simulink model "modelcomplet"  (R2021b)
settings: Solver=ode1  StartTime=0.0  StopTime=50  FixedStep=0.01  RelTol=1e-6  EnableMultiTasking=on
values from neighbouring files (symbols this model uses):
  a = -l^2+J/(mc+mp)    (= 0.00589092533208)    [parameters.m]    (also in simulation_models.m)
  A1 = expm(A(2:4,2:4)*0.01)    [simulation_models.m]
  B1 = (A1-eye(3))*inv(A(2:4,2:4))*B(2:4)    [simulation_models.m]
  DZcp = 6.8    [parameters.m]    (also in simulation_models.m)
  DZcv = 0.08    [parameters.m]    (also in simulation_models.m)
  DZu = 0.4    [parameters.m]    (also in simulation_models.m)
  FCD = 0.2501    [parameters.m]    (also in simulation_models.m)
  FCU = 0.8793    [parameters.m]    (also in simulation_models.m)
  fp = 0.0038    [parameters.m]    (also in simulation_models.m)
  FS = 2    [parameters.m]    (also in simulation_models.m)
  FSD = 2.7457    [parameters.m]    (also in simulation_models.m)
  FSdl = -1    [parameters.m]    (also in simulation_models.m)
  FSU = 2.7972    [parameters.m]    (also in simulation_models.m)
  FSul = 2    [parameters.m]    (also in simulation_models.m)
  g = 9.81    [parameters.m]    (also in simulation_models.m)
  J = 0.0075    [parameters.m]    (also in simulation_models.m)
  l = 0.0167903    [parameters.m]    (also in simulation_models.m)
  L1 = L1'    [simulation_models.m]
  M = 22.304    [parameters.m]    (also in simulation_models.m)
  mu = l*(mc+mp)    (= 0.0204002145)    [parameters.m]    (also in simulation_models.m)
  Um = 0.5    [parameters.m]    (also in simulation_models.m)
  Xc = 2    [parameters.m]    (also in simulation_models.m)
  Yc = 2    [parameters.m]    (also in simulation_models.m)
undefined symbols (not defined in the file or in its folder): DiscIntNeverNeededParam
settings Model: Creator=szmis  LastModifiedBy=szmis
settings DataIOCC: SaveFormat=Array  SignalLoggingSaveFormat=ModelDataLogs  ReturnWorkspaceOutputs=off
settings OptimizationCC: BlockReduction=off  BooleanDataType=off
settings DebuggingCC: SaveWithParameterizedLinksMsg=none  UnderspecifiedInitializationDetection=Classic  MergeDetectMultiDrivingBlocksExec=none  SignalResolutionControl=TryResolveAllWithWarning  MultiTaskDSMMsg=warning  MultiTaskCondExecSysMsg=none
settings HardwareCC: TargetUnknown=on
settings ModelReferenceCC: PropagateSignalLabelsOutOfModel=off
settings GRTTargetCC: CombineOutputUpdateFcns=off  GRTInterface=on

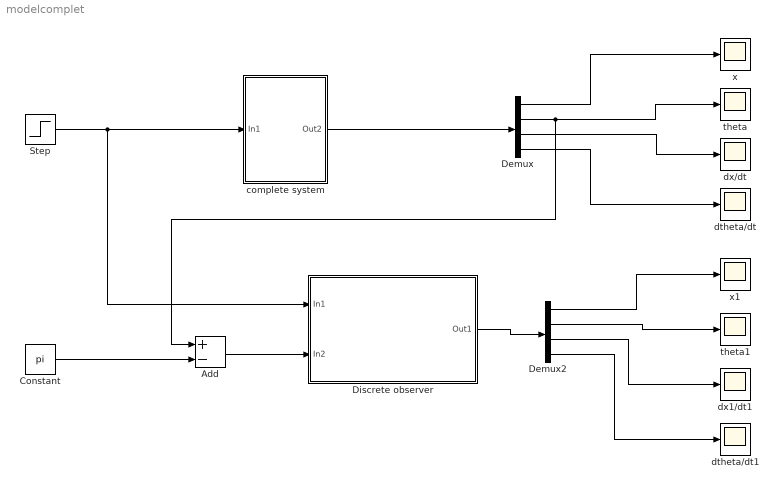
== system modelcomplet ==
  Add : Sum  Inputs=+-
  Constant : Constant  Value=pi
  Demux : Demux
  Demux2 : Demux
  Discrete observer : Subsystem
  Step : Step  After=0.3  SampleTime=0
  complete system : Subsystem
  dtheta/dt : Scope
  dtheta/dt1 : Scope
  dx/dt : Scope
  dx1/dt1 : Scope
  theta : Scope
  theta1 : Scope
  x : Scope
  x1 : Scope
  wires:
  Demux2/3 -> dx1/dt1/1
  Demux2/2 -> theta1/1
  Add/1 -> Discrete observer/2(In2)
  Demux/2 -> theta/1, Add/1
  Discrete observer/1(Out1) -> Demux2/1
  Constant/1 -> Add/2
  Demux/3 -> dx/dt/1
  Demux/1 -> x/1
  complete system/1(Out2) -> Demux/1
  Demux/4 -> dtheta/dt/1
  Demux2/1 -> x1/1
  Step/1 -> complete system/1(In1), Discrete observer/1(In1)
  Demux2/4 -> dtheta/dt1/1

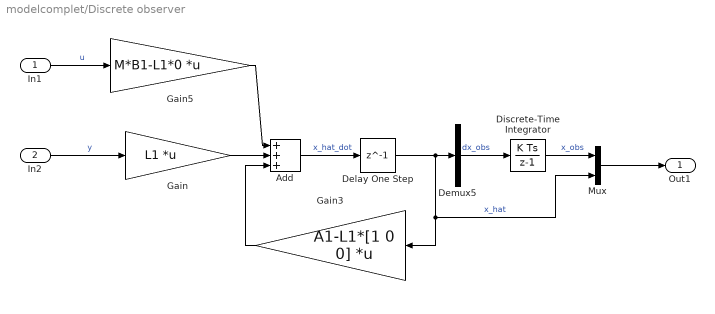
== system modelcomplet/Discrete observer ==
  In1 : Inport
  In2 : Inport  Port=2
  Add : Sum  Inputs=+++
  Delay One Step : Delay  DelayLength=1
  Demux5 : Demux  Outputs=3
  Discrete-Time Integrator : DiscreteIntegrator  SampleTime=0.01  ICPrevOutput=DiscIntNeverNeededParam  ICPrevScaledInput=DiscIntNeverNeededParam
  Gain : Gain  Gain=L1  Multiplication=Matrix(K*u)
  Gain3 : Gain  Gain=A1-L1*[1 0 0]  Multiplication=Matrix(K*u)
  Gain5 : Gain  Gain=M*B1-L1*0  Multiplication=Matrix(K*u)
  Mux : Mux  Inputs=2
  Out1 : Outport
  wires:
  In2/1 -> Gain/1  "y"
  Add/1 -> Delay One Step/1  "x_hat_dot"
  In1/1 -> Gain5/1  "u"
  Gain/1 -> Add/2
  Gain3/1 -> Add/3
  Gain5/1 -> Add/1
  Delay One Step/1 -> Demux5/1, Gain3/1, Mux/2  "x_hat"
  Mux/1 -> Out1/1
  Discrete-Time Integrator/1 -> Mux/1  "x_obs"
  Demux5/2 -> Discrete-Time Integrator/1  "dx_obs"

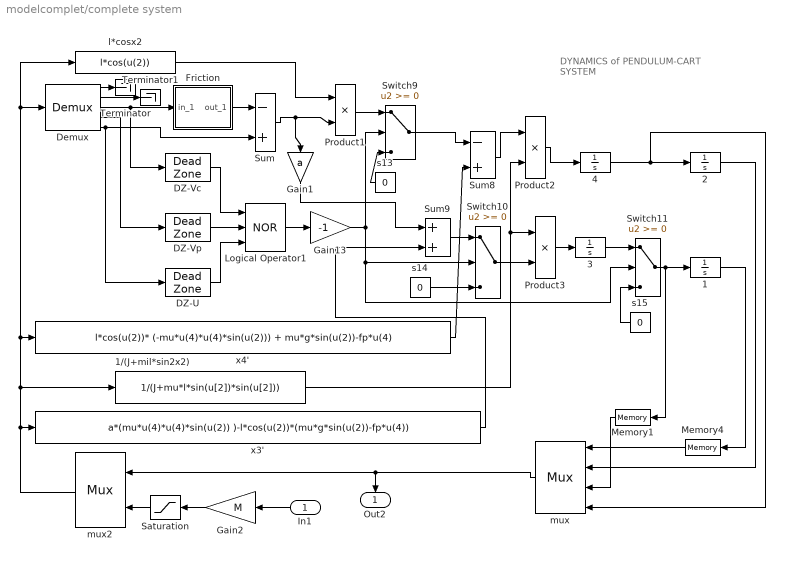
== system modelcomplet/complete system ==
  note: DYNAMICS
      | of
      | PENDULUM-CART SYSTEM
  In1 : Inport
  1 : Integrator
  1/(J+mil*sin2x2) : Fcn  Expr=1/(J+mu*l*sin(u[2])*sin(u[2]))
  2 : Integrator  InitialCondition=pi
  3 : Integrator
  4 : Integrator
  DZ-U : DeadZone  LowerValue=-DZu  UpperValue=DZu  SaturateOnIntegerOverflow=on
  DZ-Vc : DeadZone  LowerValue=-DZcv  UpperValue=DZcv  SaturateOnIntegerOverflow=on
  DZ-Vp : DeadZone  LowerValue=-DZcp  UpperValue=DZcp  SaturateOnIntegerOverflow=on
  Demux : Demux  Outputs=5
  Friction : Subsystem  mask(Friction model){FSD=FSD, FSU=FSU, FCD=FCD, FCU=FCU, FSdl=FSdl, FSul=FSul, FS=FS, Xc=Xc, Yc=Yc, small=DZcv}
      mask prompts: FSD "Static friction (FSD) [N]:"; FSU "Static friction (FSU) [N] :"; FCD "Columbic friction (FCD) [N]:"; FCU "Coulombic friction (FCU)  [N] :"; FSdl "Coulombic friction (FSdl) [N]:"; FSul "Coulombic friction (Fsul) [N]:"; FS "Coulombic friction (FS) [N]:"; Xc "Point for minimum (X1) [m/s] :"; Yc "Friction value for Xc point (Yc) [N] :"; small "Linear zone :"
      mask help: Friction implemented as nonlinear function. Copyright Adam PI�AT 1997.
      mask init:
      | Z=small;
      mask Help: Friction vs. cart velocity
      mask Display: plot(0,0,10,20,[1,9],[10,10],[5,5],[1,19],[0,1,2,3,4,5],[7,7.5,8,8.5,8.3,3],[5,6,7,8,9,10],[17,11.7,11.5,12,12.5,13])
  Gain1 : Gain  Gain=a  SaturateOnIntegerOverflow=on
  Gain13 : Gain  Gain=-1  SaturateOnIntegerOverflow=on
  Gain2 : Gain  Gain=M
  Logical Operator1 : Logic  Operator=NOR  Inputs=3
  Memory1 : Memory
  Memory4 : Memory
  Product1 : Product  SaturateOnIntegerOverflow=on
  Product2 : Product  SaturateOnIntegerOverflow=on
  Product3 : Product  SaturateOnIntegerOverflow=on
  Saturation : Saturate  UpperLimit=Um*M  LowerLimit=-Um*M
  Sum : Sum  Inputs=-+  SaturateOnIntegerOverflow=on
  Sum8 : Sum  Inputs=-+  SaturateOnIntegerOverflow=on
  Sum9 : Sum  SaturateOnIntegerOverflow=on
  Switch10 : Switch  SaturateOnIntegerOverflow=on  InputSameDT=on
  Switch11 : Switch  SaturateOnIntegerOverflow=on  InputSameDT=on
  Switch9 : Switch  SaturateOnIntegerOverflow=on  InputSameDT=on
  Terminator : Terminator
  Terminator1 : Terminator
  l*cosx2 : Fcn  Expr=l*cos(u(2))
  mux : Mux
  mux2 : Mux  Inputs=[4 1]
  s13 : Constant  Value=0
  s14 : Constant  Value=0
  s15 : Constant  Value=0
  x3' : Fcn  Expr=a*(mu*u(4)*u(4)*sin(u(2)) )-l*cos(u(2))*(mu*g*sin(u(2))-fp*u(4))
  x4' : Fcn  Expr=l*cos(u(2))* (-mu*u(4)*u(4)*sin(u(2))) + mu*g*sin(u(2))-fp*u(4)
  Out2 : Outport
  wires:
  Demux/2 -> Terminator1/1
  Demux/1 -> Terminator/1
  l*cosx2/1 -> Product1/1
  DZ-U/1 -> Logical Operator1/3
  DZ-Vp/1 -> Logical Operator1/2
  DZ-Vc/1 -> Logical Operator1/1
  Logical Operator1/1 -> Gain13/1
  s13/1 -> Switch9/3
  Switch9/1 -> Sum8/1
  s14/1 -> Switch10/3
  Product1/1 -> Switch9/1
  x4'/1 -> Sum8/2
  Sum8/1 -> Product2/1
  Product2/1 -> 4/1
  Product3/1 -> 3/1
  Demux/3 -> Friction/1(in_1), DZ-Vc/1
  Demux/4 -> DZ-Vp/1
  Sum9/1 -> Switch10/1
  s15/1 -> Switch11/3
  Memory1/1 -> mux/3
  Switch11/1 -> 1/1, Memory1/1
  Saturation/1 -> mux2/2
  Gain2/1 -> Saturation/1
  Friction/1(out_1) -> Sum/1
  Gain13/1 -> Switch9/2, Switch11/2, Switch10/2
  Demux/5 -> Sum/2, DZ-U/1
  Switch10/1 -> Product3/2
  Sum/1 -> Product1/2, Gain1/1
  Gain1/1 -> Sum9/1
  mux2/1 -> x3'/1, l*cosx2/1, Demux/1, x4'/1, 1/(J+mil*sin2x2)/1
  x3'/1 -> Sum9/2
  1/(J+mil*sin2x2)/1 -> Product2/2, Product3/1
  1/1 -> Memory4/1
  Memory4/1 -> mux/1
  4/1 -> 2/1, mux/4
  3/1 -> Switch11/1
  In1/1 -> Gain2/1
  mux/1 -> mux2/1, Out2/1
  2/1 -> mux/2

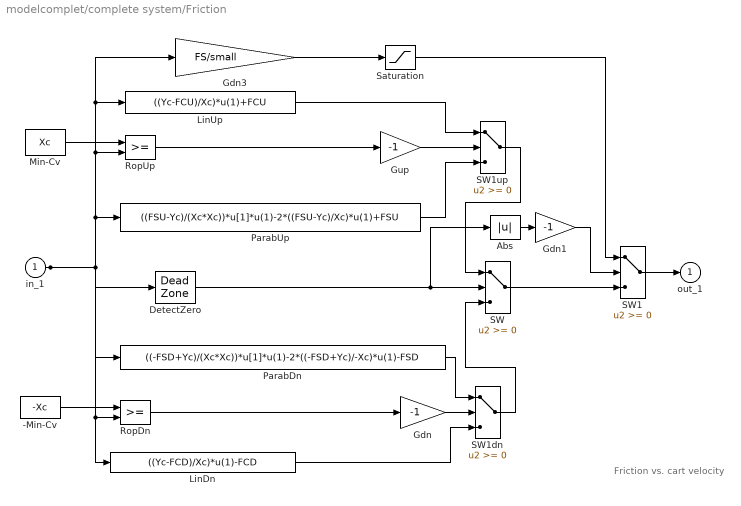
== system modelcomplet/complete system/Friction ==
  note: Friction vs. cart velocity
  in_1 : Inport
  -Min-Cv : Constant  Value=-Xc
  Abs : Abs  SaturateOnIntegerOverflow=on
  DetectZero : DeadZone  LowerValue=-Z  UpperValue=Z  SaturateOnIntegerOverflow=on
  Gdn : Gain  Gain=-1  SaturateOnIntegerOverflow=on
  Gdn1 : Gain  Gain=-1  SaturateOnIntegerOverflow=on
  Gdn3 : Gain  Gain=FS/small  SaturateOnIntegerOverflow=on
  Gup : Gain  Gain=-1  SaturateOnIntegerOverflow=on
  LinDn : Fcn  Expr=((Yc-FCD)/Xc)*u(1)-FCD
  LinUp : Fcn  Expr=((Yc-FCU)/Xc)*u(1)+FCU
  Min-Cv : Constant  Value=Xc
  ParabDn : Fcn  Expr=((-FSD+Yc)/(Xc*Xc))*u[1]*u(1)-2*((-FSD+Yc)/-Xc)*u(1)-FSD
  ParabUp : Fcn  Expr=((FSU-Yc)/(Xc*Xc))*u[1]*u(1)-2*((FSU-Yc)/Xc)*u(1)+FSU
  RopDn : RelationalOperator  RndMeth=Nearest  InputSameDT=on
  RopUp : RelationalOperator  RndMeth=Nearest  InputSameDT=on
  SW : Switch  SaturateOnIntegerOverflow=on  InputSameDT=on
  SW1 : Switch  SaturateOnIntegerOverflow=on  InputSameDT=on
  SW1dn : Switch  SaturateOnIntegerOverflow=on  InputSameDT=on
  SW1up : Switch  SaturateOnIntegerOverflow=on  InputSameDT=on
  Saturation : Saturate  UpperLimit=FSul  LowerLimit=FSdl
  out_1 : Outport  InitialOutput=0
  wires:
  Saturation/1 -> SW1/1
  Gdn3/1 -> Saturation/1
  in_1/1 -> RopUp/2, LinUp/1, Gdn3/1, ParabUp/1, ParabDn/1, DetectZero/1, LinDn/1, RopDn/2
  SW1/1 -> out_1/1
  DetectZero/1 -> SW/2, Abs/1
  Gdn1/1 -> SW1/2
  Abs/1 -> Gdn1/1
  SW/1 -> SW1/3
  Min-Cv/1 -> RopUp/1
  RopUp/1 -> Gup/1
  Gup/1 -> SW1up/2
  ParabUp/1 -> SW1up/3
  LinUp/1 -> SW1up/1
  SW1up/1 -> SW/1
  -Min-Cv/1 -> RopDn/1
  RopDn/1 -> Gdn/1
  Gdn/1 -> SW1dn/2
  LinDn/1 -> SW1dn/3
  ParabDn/1 -> SW1dn/1
  SW1dn/1 -> SW/3
